simulink model "EHB_speedgoat_R2020a_V1"  (R2020a)
settings: Solver=FixedStepDiscrete  StartTime=0.0  StopTime=inf  FixedStep=0.001  RelTol=1e-3  EnableMultiTasking=on
model workspace (MAT data in the model file):
  A : Simulink.Signal (value not decoded)
  B : Simulink.Signal (value not decoded)
  C : Simulink.Signal (value not decoded)
  D : Simulink.Signal (value not decoded)
  E : Simulink.Signal (value not decoded)
  calin = [-9.96 -7.98 -5.98 -3.99 -1.994 0 1.995 3.992 5.99 7.98 9.97]
  calout = [-10 -8 -6 -4 -2 0 2 4 6 8 10]
symbols that are objects in the model workspace (value not decoded): C, D
undefined symbols (not defined in the file): Com1, none, ts_IO612
libraries: simulink x1436, xpcethercatlib x1223, yisutbxlib_utilities x256, xpcutilitieslib x156, hdlsllib x145, canmsglib x46, speedgoatlib_IO602_4 x11, speedgoatlib_IO611 x7, slrttcplib x4, CanManageLib x3, slrtlib x3, xpcseriallib x2
(part 25 of 30)

== system EHB_speedgoat_R2020a_V1/保留/YS4008/YS4008_M_5/YS4008_M/FIU_MsgSend ==
  YS4008_M : Inport
  Enable : EnablePort
  Bus Selector : BusSelector  OutputSignals=CH1_Out.KL30_Out,CH1_Out.KL31_Out,CH1_Out.COM_Out,CH1_Out.Open_Out,CH2_Out.KL30_Out,CH2_Out.KL31_Out,CH2_Out.COM_Out,CH2_Out.Open_Out,CH3_Out.KL30_Out,CH3_Out.KL31_Out,CH3_Out.COM_Out,CH3_Out.Open_Out,CH4_Out.KL30_Out,CH4_Out.KL31_Out,CH4_Out.COM_Out,CH4_Out.Open_Out,CH5_Out.KL30_Out,CH5_Out.KL31_Out,CH5_Out.COM_Out,CH5_Out.Open_Out,CH6_Out.KL30_Out,CH6_Out.KL31_Out,CH6_Out.COM_Out,CH6_Out.Open_Out,CH7_Out.KL30_Out,CH7_Out.KL31_Out,CH7_Out.COM_Out,CH7_Out.Open_Out,CH8_Out.KL30_Out,CH8_Out.KL31_Out,CH8_Out.COM_Out,CH8_Out.Open_Out,PassWord,Rack,Slot
  CAN Pack8 : canmsglib/CAN Pack  MsgList=(none)  MsgName=FIUStsSet  MsgIDType=Standard (11-bit identifier)  MsgIdentifier=1669  MsgLength=8  Remote=off  ApplyMinMax=off  BusOutput=on  SignalInfo={ 'CH1_COM', '26', '1', 'BE', 'unsigned', 'Standard', '0', '1', '0', '0', '1'; 'CH1_KL30', '24', '1', 'BE', 'unsigned', 'Standard', '0', '1', '0', '0', '1'; 'CH1_KL31', '25', '1', 'BE', 'unsigned', 'Standard', '0', '1', '0', '0', '1'; 'CH1_Open', '27', '1', 'BE', 'unsigned', 'Standard', '0', '1', '0', '0', '1'; 'CH2_COM', '30', '1', 'BE', 'unsigned', 'Standard', '0', '1', '0', '0', '1'; 'CH2_KL30', '28', '1', 'BE', 'unsigned', 'Standard', '0', '1', '0', '0', '1'; 'CH2_KL31', '29', '1', 'BE', 'unsigned', 'Standard', '0', '1', '0', '0', '1'; 'CH2_Open', '31', '1', 'BE', 'unsigned', 'Standard', '0', '1', '0', '0', '1'; 'CH3_COM', '34', '1', 'BE', 'unsigned', 'Standard', '0', '1', '0', '0', '1'; 'CH3_KL30', '32', '1', 'BE', 'unsigned', 'Standard', '0', '1', '0', '0', '1'; 'CH3_KL31', '33', '1', 'BE', 'unsigned', 'Standard', '0', '1', '0', '0', '1'; 'CH3_Open', '35', '1', 'BE', 'unsigned', 'Standard', '0', '1', '0', '0', '1'; 'CH4_COM', '38', '1', 'BE', 'unsigned', 'Standard', '0', '1', '0', '0', '1'; 'CH4_KL30', '36', '1', 'BE', 'unsigned', 'Standard', '0', '1', '0', '0', '1'; 'CH4_KL31', '37', '1', 'BE', 'unsigned', 'Standard', '0', '1', '0', '0', '1'; 'CH4_Open', '39', '1', 'BE', 'unsigned', 'Standard', '0', '1', '0', '0', '1'; 'CH5_COM', '42', '1', 'BE', 'unsigned', 'Standard', '0', '1', '0', '0', '1'; 'CH5_KL30', '40', '1', 'BE', 'unsigned', 'Standard', '0', '1', '0', '0', '1'; 'CH5_KL31', '41', '1', 'BE', 'unsigned', 'Standard', '0', '1', '0', '0', '1'; 'CH5_Open', '43', '1', 'BE', 'unsigned', 'Standard', '0', '1', '0', '0', '1'; 'CH6_COM', '46', '1', 'BE', 'unsigned', 'Standard', '0', '1', '0', '0', '1'; 'CH6_KL30', '44', '1', 'BE', 'unsigned', 'Standard', '0', '1', '0', '0', '1'; 'CH6_KL31', '45', '1', 'BE', 'unsigned', 'Standard', '0', '1', '0', '0', '1'; 'CH6_Open', '47', '1', 'BE', 'unsigned', 'Standard', '0', '1', '0', '0', '1'; 'CH7_COM', '50', '1', 'BE', 'unsigned', 'Standard', '0', '1', '0', '0', '1'; 'CH7_KL30', '48', '1', 'BE', 'unsigned', 'Standard', '0', '1', '0', '0', '1'; 'CH7_KL31', '49', '1', 'BE', 'unsigned', 'Standard', '0', '1', '0', '0', '1'; 'CH7_Open', '51', '1', 'BE', 'unsigned', 'Standard', '0', '1', '0', '0', '1'; 'CH8_COM', '54', '1', 'BE', 'unsigned', 'Standard', '0', '1', '0', '0', '1'; 'CH8_KL30', '52', '1', 'BE', 'unsigned', 'Standard', '0', '1', '0', '0', '1'; 'CH8_KL31', '53', '1', 'BE', 'unsigned', 'Standard', '0', '1', '0', '0', '1'; 'CH8_Open', '55', '1', 'BE', 'unsigned', 'Standard', '0', '1', '0', '0', '1'; 'Password', '16', '8', 'BE', 'unsigned', 'Standard', '0', '1', '0', '0', '15'; 'Rack', '0', '4', 'BE', 'signed', 'Standard', '0', '1', '0', '-Inf', 'Inf'; 'Slot', '4', '4', 'BE', 'signed', 'Standard', '0', '1', '0', '-Inf', 'Inf' }
      settings: SourceProductBaseCode=XP,ME,VN  DataFormat=manually specified signals
  CANDataPack_ToUDP : Subsystem
  Output : Outport
  wires:
  YS4008_M/1 -> Bus Selector/1
  [CH1_COM] -> CAN Pack8/1  "CH1_COM"
  [CH1_KL30] -> CAN Pack8/2  "CH1_KL30"
  [CH1_KL31] -> CAN Pack8/3  "CH1_KL31"
  [CH1_Open] -> CAN Pack8/4  "CH1_Open"
  [CH2_COM] -> CAN Pack8/5  "CH2_COM"
  [CH2_KL30] -> CAN Pack8/6  "CH2_KL30"
  [CH2_KL31] -> CAN Pack8/7  "CH2_KL31"
  [CH2_Open] -> CAN Pack8/8  "CH2_Open"
  [CH3_COM] -> CAN Pack8/9  "CH3_COM"
  [CH3_KL30] -> CAN Pack8/10  "CH3_KL30"
  [CH3_KL31] -> CAN Pack8/11  "CH3_KL31"
  [CH3_Open] -> CAN Pack8/12  "CH3_Open"
  [CH4_COM] -> CAN Pack8/13  "CH4_COM"
  [CH4_KL30] -> CAN Pack8/14  "CH4_KL30"
  [CH4_KL31] -> CAN Pack8/15  "CH4_KL31"
  [CH4_Open] -> CAN Pack8/16  "CH4_Open"
  [CH5_COM] -> CAN Pack8/17  "CH5_COM"
  [CH5_KL30] -> CAN Pack8/18  "CH5_KL30"
  [CH5_KL31] -> CAN Pack8/19  "CH5_KL31"
  [CH5_Open] -> CAN Pack8/20  "CH5_Open"
  [CH6_COM] -> CAN Pack8/21  "CH6_COM"
  [CH6_KL30] -> CAN Pack8/22  "CH6_KL30"
  [CH6_KL31] -> CAN Pack8/23  "CH6_KL31"
  [CH6_Open] -> CAN Pack8/24  "CH6_Open"
  [CH7_COM] -> CAN Pack8/25  "CH7_COM"
  [CH7_KL30] -> CAN Pack8/26  "CH7_KL30"
  [CH7_KL31] -> CAN Pack8/27  "CH7_KL31"
  [CH7_Open] -> CAN Pack8/28  "CH7_Open"
  [CH8_COM] -> CAN Pack8/29  "CH8_COM"
  [CH8_KL30] -> CAN Pack8/30  "CH8_KL30"
  [CH8_KL31] -> CAN Pack8/31  "CH8_KL31"
  [CH8_Open] -> CAN Pack8/32  "CH8_Open"
  [PassWord] -> CAN Pack8/33  "PassWord"
  Bus Selector/33 -> [PassWord]  "<PassWord>"
  Bus Selector/9 -> [CH3_KL30]  "<KL30_Out>"
  Bus Selector/10 -> [CH3_KL31]  "<KL31_Out>"
  Bus Selector/11 -> [CH3_COM]  "<COM_Out>"
  Bus Selector/12 -> [CH3_Open]  "<Open_Out>"
  Bus Selector/13 -> [CH4_KL30]  "<KL30_Out>"
  Bus Selector/14 -> [CH4_KL31]  "<KL31_Out>"
  Bus Selector/15 -> [CH4_COM]  "<COM_Out>"
  Bus Selector/16 -> [CH4_Open]  "<Open_Out>"
  Bus Selector/17 -> [CH5_KL30]  "<KL30_Out>"
  Bus Selector/18 -> [CH5_KL31]  "<KL31_Out>"
  Bus Selector/19 -> [CH5_COM]  "<COM_Out>"
  Bus Selector/20 -> [CH5_Open]  "<Open_Out>"
  Bus Selector/21 -> [CH6_KL30]  "<KL30_Out>"
  Bus Selector/22 -> [CH6_KL31]  "<KL31_Out>"
  Bus Selector/23 -> [CH6_COM]  "<COM_Out>"
  Bus Selector/24 -> [CH6_Open]  "<Open_Out>"
  Bus Selector/25 -> [CH7_KL30]  "<KL30_Out>"
  Bus Selector/26 -> [CH7_KL31]  "<KL31_Out>"
  Bus Selector/27 -> [CH7_COM]  "<COM_Out>"
  Bus Selector/28 -> [CH7_Open]  "<Open_Out>"
  Bus Selector/29 -> [CH8_KL30]  "<KL30_Out>"
  Bus Selector/30 -> [CH8_KL31]  "<KL31_Out>"
  Bus Selector/31 -> [CH8_COM]  "<COM_Out>"
  Bus Selector/32 -> [CH8_Open]  "<Open_Out>"
  Bus Selector/1 -> [CH1_KL30]  "<KL30_Out>"
  Bus Selector/2 -> [CH1_KL31]  "<KL31_Out>"
  Bus Selector/3 -> [CH1_COM]  "<COM_Out>"
  Bus Selector/4 -> [CH1_Open]  "<Open_Out>"
  Bus Selector/5 -> [CH2_KL30]  "<KL30_Out>"
  Bus Selector/6 -> [CH2_KL31]  "<KL31_Out>"
  Bus Selector/7 -> [CH2_COM]  "<COM_Out>"
  Bus Selector/8 -> [CH2_Open]  "<Open_Out>"
  [Rack] -> CAN Pack8/34  "Rack"
  [Slot] -> CAN Pack8/35  "Slot"
  Bus Selector/34 -> [Rack]  "<Rack>"
  Bus Selector/35 -> [Slot]  "<Slot>"
  CAN Pack8/1 -> CANDataPack_ToUDP/1(In1)
  CANDataPack_ToUDP/1(Output) -> Output/1

== system EHB_speedgoat_R2020a_V1/保留/YS4008/YS4008_M_5/YS4008_M/YS4008_M_Ctrl_Trigger ==
  YS4008_M : Inport
  Bitwise Operator : simulink/Logic and Bit Operations/Bitwise Operator  logicop=OR  UseBitMask=off  BitMask=bin2dec('11011001')  BitMaskRealWorld=Stored Integer
  Bus Selector : BusSelector  OutputSignals=FIU_SetCH1,FIU_SetCH2,FIU_SetCH3,FIU_SetCH4,FIU_SetCH5,FIU_SetCH6,FIU_SetCH7,FIU_SetCH8
  Detect Change : simulink/Logic and Bit Operations/Detect Change  vinit=0  OutDataTypeStr=boolean
  Mux : Mux  Inputs=8
  YS4008_M_CtrlTrigger : Outport
  wires:
  Detect Change/1 -> Bitwise Operator/1
  Mux/1 -> Detect Change/1
  Bitwise Operator/1 -> YS4008_M_CtrlTrigger/1
  YS4008_M/1 -> Bus Selector/1
  Bus Selector/1 -> Mux/1  "<FIU_SetCH1>"
  Bus Selector/2 -> Mux/2  "<FIU_SetCH2>"
  Bus Selector/3 -> Mux/3  "<FIU_SetCH3>"
  Bus Selector/4 -> Mux/4  "<FIU_SetCH4>"
  Bus Selector/5 -> Mux/5  "<FIU_SetCH5>"
  Bus Selector/6 -> Mux/6  "<FIU_SetCH6>"
  Bus Selector/7 -> Mux/7  "<FIU_SetCH7>"
  Bus Selector/8 -> Mux/8  "<FIU_SetCH8>"

== system EHB_speedgoat_R2020a_V1/保留/YS4008/YS4008_M_6/YS4008_M/FIU_CH1 ==
  FIU_SetCH1 : Inport
  Bit Unpacking 1 : xpcutilitieslib/Bit Unpacking   SignExtend=on  MaskBitPatterns={[0],[1],[2],[3]}  MaskPackDataType=uint8  MaskPackDataSize=[1]  MaskUnpackDataTypes={'boolean','boolean','boolean','boolean'}  MaskUnpackDataSizes={[1],[1],[1],[1]}
      settings: SourceProductBaseCode=XP
  Bus Creator : BusCreator  Inputs=4
  Protect : Subsystem
  CH1_Out : Outport
  wires:
  FIU_SetCH1/1 -> Bit Unpacking 1/1
  Protect/3(COM_Out) -> Bus Creator/3  "COM_Out"
  Protect/2(KL31_Out) -> Bus Creator/2  "KL31_Out"
  Protect/1(KL30_Out) -> Bus Creator/1  "KL30_Out"
  Protect/4(Open_Out) -> Bus Creator/4  "Open_Out"
  Bit Unpacking 1/1 -> Protect/1(KL30_In)
  Bit Unpacking 1/2 -> Protect/2(KL31_In)
  Bit Unpacking 1/3 -> Protect/3(COM_In)
  Bit Unpacking 1/4 -> Protect/4(Open_In)
  Bus Creator/1 -> CH1_Out/1

== system EHB_speedgoat_R2020a_V1/保留/YS4008/YS4008_M_6/YS4008_M/FIU_CH2 ==
  FIU_SetCH2 : Inport
  Bit Unpacking 1 : xpcutilitieslib/Bit Unpacking   SignExtend=on  MaskBitPatterns={[0],[1],[2],[3]}  MaskPackDataType=uint8  MaskPackDataSize=[1]  MaskUnpackDataTypes={'boolean','boolean','boolean','boolean'}  MaskUnpackDataSizes={[1],[1],[1],[1]}
      settings: SourceProductBaseCode=XP
  Bus Creator : BusCreator  Inputs=4
  Protect : Subsystem
  CH2_Out : Outport
  wires:
  Bus Creator/1 -> CH2_Out/1
  Bit Unpacking 1/4 -> Protect/4(Open_In)
  Bit Unpacking 1/3 -> Protect/3(COM_In)
  Bit Unpacking 1/2 -> Protect/2(KL31_In)
  Bit Unpacking 1/1 -> Protect/1(KL30_In)
  Protect/4(Open_Out) -> Bus Creator/4  "Open_Out"
  Protect/1(KL30_Out) -> Bus Creator/1  "KL30_Out"
  Protect/2(KL31_Out) -> Bus Creator/2  "KL31_Out"
  Protect/3(COM_Out) -> Bus Creator/3  "COM_Out"
  FIU_SetCH2/1 -> Bit Unpacking 1/1

== system EHB_speedgoat_R2020a_V1/保留/YS4008/YS4008_M_6/YS4008_M/FIU_CH3 ==
  FIU_SetCH3 : Inport
  Bit Unpacking 1 : xpcutilitieslib/Bit Unpacking   SignExtend=on  MaskBitPatterns={[0],[1],[2],[3]}  MaskPackDataType=uint8  MaskPackDataSize=[1]  MaskUnpackDataTypes={'boolean','boolean','boolean','boolean'}  MaskUnpackDataSizes={[1],[1],[1],[1]}
      settings: SourceProductBaseCode=XP
  Bus Creator : BusCreator  Inputs=4
  Protect : Subsystem
  CH3_Out : Outport
  wires:
  FIU_SetCH3/1 -> Bit Unpacking 1/1
  Protect/3(COM_Out) -> Bus Creator/3  "COM_Out"
  Protect/2(KL31_Out) -> Bus Creator/2  "KL31_Out"
  Protect/1(KL30_Out) -> Bus Creator/1  "KL30_Out"
  Protect/4(Open_Out) -> Bus Creator/4  "Open_Out"
  Bit Unpacking 1/1 -> Protect/1(KL30_In)
  Bit Unpacking 1/2 -> Protect/2(KL31_In)
  Bit Unpacking 1/3 -> Protect/3(COM_In)
  Bit Unpacking 1/4 -> Protect/4(Open_In)
  Bus Creator/1 -> CH3_Out/1

== system EHB_speedgoat_R2020a_V1/保留/YS4008/YS4008_M_6/YS4008_M/FIU_CH4 ==
  FIU_SetCH4 : Inport
  Bit Unpacking 1 : xpcutilitieslib/Bit Unpacking   SignExtend=on  MaskBitPatterns={[0],[1],[2],[3]}  MaskPackDataType=uint8  MaskPackDataSize=[1]  MaskUnpackDataTypes={'boolean','boolean','boolean','boolean'}  MaskUnpackDataSizes={[1],[1],[1],[1]}
      settings: SourceProductBaseCode=XP
  Bus Creator : BusCreator  Inputs=4
  Protect : Subsystem
  CH4_Out : Outport
  wires:
  Bus Creator/1 -> CH4_Out/1
  Bit Unpacking 1/4 -> Protect/4(Open_In)
  Bit Unpacking 1/3 -> Protect/3(COM_In)
  Bit Unpacking 1/2 -> Protect/2(KL31_In)
  Bit Unpacking 1/1 -> Protect/1(KL30_In)
  Protect/4(Open_Out) -> Bus Creator/4  "Open_Out"
  Protect/1(KL30_Out) -> Bus Creator/1  "KL30_Out"
  Protect/2(KL31_Out) -> Bus Creator/2  "KL31_Out"
  Protect/3(COM_Out) -> Bus Creator/3  "COM_Out"
  FIU_SetCH4/1 -> Bit Unpacking 1/1

== system EHB_speedgoat_R2020a_V1/保留/YS4008/YS4008_M_6/YS4008_M/FIU_CH5 ==
  FIU_SetCH5 : Inport
  Bit Unpacking 1 : xpcutilitieslib/Bit Unpacking   SignExtend=on  MaskBitPatterns={[0],[1],[2],[3]}  MaskPackDataType=uint8  MaskPackDataSize=[1]  MaskUnpackDataTypes={'boolean','boolean','boolean','boolean'}  MaskUnpackDataSizes={[1],[1],[1],[1]}
      settings: SourceProductBaseCode=XP
  Bus Creator : BusCreator  Inputs=4
  Protect : Subsystem
  CH5_Out : Outport
  wires:
  FIU_SetCH5/1 -> Bit Unpacking 1/1
  Protect/3(COM_Out) -> Bus Creator/3  "COM_Out"
  Protect/2(KL31_Out) -> Bus Creator/2  "KL31_Out"
  Protect/1(KL30_Out) -> Bus Creator/1  "KL30_Out"
  Protect/4(Open_Out) -> Bus Creator/4  "Open_Out"
  Bit Unpacking 1/1 -> Protect/1(KL30_In)
  Bit Unpacking 1/2 -> Protect/2(KL31_In)
  Bit Unpacking 1/3 -> Protect/3(COM_In)
  Bit Unpacking 1/4 -> Protect/4(Open_In)
  Bus Creator/1 -> CH5_Out/1

== system EHB_speedgoat_R2020a_V1/保留/YS4008/YS4008_M_6/YS4008_M/FIU_CH6 ==
  FIU_SetCH6 : Inport
  Bit Unpacking 1 : xpcutilitieslib/Bit Unpacking   SignExtend=on  MaskBitPatterns={[0],[1],[2],[3]}  MaskPackDataType=uint8  MaskPackDataSize=[1]  MaskUnpackDataTypes={'boolean','boolean','boolean','boolean'}  MaskUnpackDataSizes={[1],[1],[1],[1]}
      settings: SourceProductBaseCode=XP
  Bus Creator : BusCreator  Inputs=4
  Protect : Subsystem
  CH6_Out : Outport
  wires:
  Bus Creator/1 -> CH6_Out/1
  Bit Unpacking 1/4 -> Protect/4(Open_In)
  Bit Unpacking 1/3 -> Protect/3(COM_In)
  Bit Unpacking 1/2 -> Protect/2(KL31_In)
  Bit Unpacking 1/1 -> Protect/1(KL30_In)
  Protect/4(Open_Out) -> Bus Creator/4  "Open_Out"
  Protect/1(KL30_Out) -> Bus Creator/1  "KL30_Out"
  Protect/2(KL31_Out) -> Bus Creator/2  "KL31_Out"
  Protect/3(COM_Out) -> Bus Creator/3  "COM_Out"
  FIU_SetCH6/1 -> Bit Unpacking 1/1

== system EHB_speedgoat_R2020a_V1/保留/YS4008/YS4008_M_6/YS4008_M/FIU_CH7 ==
  FIU_SetCH7 : Inport
  Bit Unpacking 1 : xpcutilitieslib/Bit Unpacking   SignExtend=on  MaskBitPatterns={[0],[1],[2],[3]}  MaskPackDataType=uint8  MaskPackDataSize=[1]  MaskUnpackDataTypes={'boolean','boolean','boolean','boolean'}  MaskUnpackDataSizes={[1],[1],[1],[1]}
      settings: SourceProductBaseCode=XP
  Bus Creator : BusCreator  Inputs=4
  Protect : Subsystem
  CH7_Out : Outport
  wires:
  FIU_SetCH7/1 -> Bit Unpacking 1/1
  Protect/3(COM_Out) -> Bus Creator/3  "COM_Out"
  Protect/2(KL31_Out) -> Bus Creator/2  "KL31_Out"
  Protect/1(KL30_Out) -> Bus Creator/1  "KL30_Out"
  Protect/4(Open_Out) -> Bus Creator/4  "Open_Out"
  Bit Unpacking 1/1 -> Protect/1(KL30_In)
  Bit Unpacking 1/2 -> Protect/2(KL31_In)
  Bit Unpacking 1/3 -> Protect/3(COM_In)
  Bit Unpacking 1/4 -> Protect/4(Open_In)
  Bus Creator/1 -> CH7_Out/1

== system EHB_speedgoat_R2020a_V1/保留/YS4008/YS4008_M_6/YS4008_M/FIU_CH8 ==
  FIU_SetCH8 : Inport
  Bit Unpacking 1 : xpcutilitieslib/Bit Unpacking   SignExtend=on  MaskBitPatterns={[0],[1],[2],[3]}  MaskPackDataType=uint8  MaskPackDataSize=[1]  MaskUnpackDataTypes={'boolean','boolean','boolean','boolean'}  MaskUnpackDataSizes={[1],[1],[1],[1]}
      settings: SourceProductBaseCode=XP
  Bus Creator : BusCreator  Inputs=4
  Protect : Subsystem
  CH8_Out : Outport
  wires:
  Bus Creator/1 -> CH8_Out/1
  Bit Unpacking 1/4 -> Protect/4(Open_In)
  Bit Unpacking 1/3 -> Protect/3(COM_In)
  Bit Unpacking 1/2 -> Protect/2(KL31_In)
  Bit Unpacking 1/1 -> Protect/1(KL30_In)
  Protect/4(Open_Out) -> Bus Creator/4  "Open_Out"
  Protect/1(KL30_Out) -> Bus Creator/1  "KL30_Out"
  Protect/2(KL31_Out) -> Bus Creator/2  "KL31_Out"
  Protect/3(COM_Out) -> Bus Creator/3  "COM_Out"
  FIU_SetCH8/1 -> Bit Unpacking 1/1

== system EHB_speedgoat_R2020a_V1/保留/YS4008/YS4008_M_6/YS4008_M/FIU_MsgSend ==
  YS4008_M : Inport
  Enable : EnablePort
  Bus Selector : BusSelector  OutputSignals=CH1_Out.KL30_Out,CH1_Out.KL31_Out,CH1_Out.COM_Out,CH1_Out.Open_Out,CH2_Out.KL30_Out,CH2_Out.KL31_Out,CH2_Out.COM_Out,CH2_Out.Open_Out,CH3_Out.KL30_Out,CH3_Out.KL31_Out,CH3_Out.COM_Out,CH3_Out.Open_Out,CH4_Out.KL30_Out,CH4_Out.KL31_Out,CH4_Out.COM_Out,CH4_Out.Open_Out,CH5_Out.KL30_Out,CH5_Out.KL31_Out,CH5_Out.COM_Out,CH5_Out.Open_Out,CH6_Out.KL30_Out,CH6_Out.KL31_Out,CH6_Out.COM_Out,CH6_Out.Open_Out,CH7_Out.KL30_Out,CH7_Out.KL31_Out,CH7_Out.COM_Out,CH7_Out.Open_Out,CH8_Out.KL30_Out,CH8_Out.KL31_Out,CH8_Out.COM_Out,CH8_Out.Open_Out,PassWord,Rack,Slot
  CAN Pack8 : canmsglib/CAN Pack  MsgList=(none)  MsgName=FIUStsSet  MsgIDType=Standard (11-bit identifier)  MsgIdentifier=1670  MsgLength=8  Remote=off  ApplyMinMax=off  BusOutput=on  SignalInfo={ 'CH1_COM', '26', '1', 'BE', 'unsigned', 'Standard', '0', '1', '0', '0', '1'; 'CH1_KL30', '24', '1', 'BE', 'unsigned', 'Standard', '0', '1', '0', '0', '1'; 'CH1_KL31', '25', '1', 'BE', 'unsigned', 'Standard', '0', '1', '0', '0', '1'; 'CH1_Open', '27', '1', 'BE', 'unsigned', 'Standard', '0', '1', '0', '0', '1'; 'CH2_COM', '30', '1', 'BE', 'unsigned', 'Standard', '0', '1', '0', '0', '1'; 'CH2_KL30', '28', '1', 'BE', 'unsigned', 'Standard', '0', '1', '0', '0', '1'; 'CH2_KL31', '29', '1', 'BE', 'unsigned', 'Standard', '0', '1', '0', '0', '1'; 'CH2_Open', '31', '1', 'BE', 'unsigned', 'Standard', '0', '1', '0', '0', '1'; 'CH3_COM', '34', '1', 'BE', 'unsigned', 'Standard', '0', '1', '0', '0', '1'; 'CH3_KL30', '32', '1', 'BE', 'unsigned', 'Standard', '0', '1', '0', '0', '1'; 'CH3_KL31', '33', '1', 'BE', 'unsigned', 'Standard', '0', '1', '0', '0', '1'; 'CH3_Open', '35', '1', 'BE', 'unsigned', 'Standard', '0', '1', '0', '0', '1'; 'CH4_COM', '38', '1', 'BE', 'unsigned', 'Standard', '0', '1', '0', '0', '1'; 'CH4_KL30', '36', '1', 'BE', 'unsigned', 'Standard', '0', '1', '0', '0', '1'; 'CH4_KL31', '37', '1', 'BE', 'unsigned', 'Standard', '0', '1', '0', '0', '1'; 'CH4_Open', '39', '1', 'BE', 'unsigned', 'Standard', '0', '1', '0', '0', '1'; 'CH5_COM', '42', '1', 'BE', 'unsigned', 'Standard', '0', '1', '0', '0', '1'; 'CH5_KL30', '40', '1', 'BE', 'unsigned', 'Standard', '0', '1', '0', '0', '1'; 'CH5_KL31', '41', '1', 'BE', 'unsigned', 'Standard', '0', '1', '0', '0', '1'; 'CH5_Open', '43', '1', 'BE', 'unsigned', 'Standard', '0', '1', '0', '0', '1'; 'CH6_COM', '46', '1', 'BE', 'unsigned', 'Standard', '0', '1', '0', '0', '1'; 'CH6_KL30', '44', '1', 'BE', 'unsigned', 'Standard', '0', '1', '0', '0', '1'; 'CH6_KL31', '45', '1', 'BE', 'unsigned', 'Standard', '0', '1', '0', '0', '1'; 'CH6_Open', '47', '1', 'BE', 'unsigned', 'Standard', '0', '1', '0', '0', '1'; 'CH7_COM', '50', '1', 'BE', 'unsigned', 'Standard', '0', '1', '0', '0', '1'; 'CH7_KL30', '48', '1', 'BE', 'unsigned', 'Standard', '0', '1', '0', '0', '1'; 'CH7_KL31', '49', '1', 'BE', 'unsigned', 'Standard', '0', '1', '0', '0', '1'; 'CH7_Open', '51', '1', 'BE', 'unsigned', 'Standard', '0', '1', '0', '0', '1'; 'CH8_COM', '54', '1', 'BE', 'unsigned', 'Standard', '0', '1', '0', '0', '1'; 'CH8_KL30', '52', '1', 'BE', 'unsigned', 'Standard', '0', '1', '0', '0', '1'; 'CH8_KL31', '53', '1', 'BE', 'unsigned', 'Standard', '0', '1', '0', '0', '1'; 'CH8_Open', '55', '1', 'BE', 'unsigned', 'Standard', '0', '1', '0', '0', '1'; 'Password', '16', '8', 'BE', 'unsigned', 'Standard', '0', '1', '0', '0', '15'; 'Rack', '0', '4', 'BE', 'signed', 'Standard', '0', '1', '0', '-Inf', 'Inf'; 'Slot', '4', '4', 'BE', 'signed', 'Standard', '0', '1', '0', '-Inf', 'Inf' }
      settings: SourceProductBaseCode=XP,ME,VN  DataFormat=manually specified signals
  CANDataPack_ToUDP : Subsystem
  Output : Outport
  wires:
  YS4008_M/1 -> Bus Selector/1
  [CH1_COM] -> CAN Pack8/1  "CH1_COM"
  [CH1_KL30] -> CAN Pack8/2  "CH1_KL30"
  [CH1_KL31] -> CAN Pack8/3  "CH1_KL31"
  [CH1_Open] -> CAN Pack8/4  "CH1_Open"
  [CH2_COM] -> CAN Pack8/5  "CH2_COM"
  [CH2_KL30] -> CAN Pack8/6  "CH2_KL30"
  [CH2_KL31] -> CAN Pack8/7  "CH2_KL31"
  [CH2_Open] -> CAN Pack8/8  "CH2_Open"
  [CH3_COM] -> CAN Pack8/9  "CH3_COM"
  [CH3_KL30] -> CAN Pack8/10  "CH3_KL30"
  [CH3_KL31] -> CAN Pack8/11  "CH3_KL31"
  [CH3_Open] -> CAN Pack8/12  "CH3_Open"
  [CH4_COM] -> CAN Pack8/13  "CH4_COM"
  [CH4_KL30] -> CAN Pack8/14  "CH4_KL30"
  [CH4_KL31] -> CAN Pack8/15  "CH4_KL31"
  [CH4_Open] -> CAN Pack8/16  "CH4_Open"
  [CH5_COM] -> CAN Pack8/17  "CH5_COM"
  [CH5_KL30] -> CAN Pack8/18  "CH5_KL30"
  [CH5_KL31] -> CAN Pack8/19  "CH5_KL31"
  [CH5_Open] -> CAN Pack8/20  "CH5_Open"
  [CH6_COM] -> CAN Pack8/21  "CH6_COM"
  [CH6_KL30] -> CAN Pack8/22  "CH6_KL30"
  [CH6_KL31] -> CAN Pack8/23  "CH6_KL31"
  [CH6_Open] -> CAN Pack8/24  "CH6_Open"
  [CH7_COM] -> CAN Pack8/25  "CH7_COM"
  [CH7_KL30] -> CAN Pack8/26  "CH7_KL30"
  [CH7_KL31] -> CAN Pack8/27  "CH7_KL31"
  [CH7_Open] -> CAN Pack8/28  "CH7_Open"
  [CH8_COM] -> CAN Pack8/29  "CH8_COM"
  [CH8_KL30] -> CAN Pack8/30  "CH8_KL30"
  [CH8_KL31] -> CAN Pack8/31  "CH8_KL31"
  [CH8_Open] -> CAN Pack8/32  "CH8_Open"
  [PassWord] -> CAN Pack8/33  "PassWord"
  Bus Selector/33 -> [PassWord]  "<PassWord>"
  Bus Selector/9 -> [CH3_KL30]  "<KL30_Out>"
  Bus Selector/10 -> [CH3_KL31]  "<KL31_Out>"
  Bus Selector/11 -> [CH3_COM]  "<COM_Out>"
  Bus Selector/12 -> [CH3_Open]  "<Open_Out>"
  Bus Selector/13 -> [CH4_KL30]  "<KL30_Out>"
  Bus Selector/14 -> [CH4_KL31]  "<KL31_Out>"
  Bus Selector/15 -> [CH4_COM]  "<COM_Out>"
  Bus Selector/16 -> [CH4_Open]  "<Open_Out>"
  Bus Selector/17 -> [CH5_KL30]  "<KL30_Out>"
  Bus Selector/18 -> [CH5_KL31]  "<KL31_Out>"
  Bus Selector/19 -> [CH5_COM]  "<COM_Out>"
  Bus Selector/20 -> [CH5_Open]  "<Open_Out>"
  Bus Selector/21 -> [CH6_KL30]  "<KL30_Out>"
  Bus Selector/22 -> [CH6_KL31]  "<KL31_Out>"
  Bus Selector/23 -> [CH6_COM]  "<COM_Out>"
  Bus Selector/24 -> [CH6_Open]  "<Open_Out>"
  Bus Selector/25 -> [CH7_KL30]  "<KL30_Out>"
  Bus Selector/26 -> [CH7_KL31]  "<KL31_Out>"
  Bus Selector/27 -> [CH7_COM]  "<COM_Out>"
  Bus Selector/28 -> [CH7_Open]  "<Open_Out>"
  Bus Selector/29 -> [CH8_KL30]  "<KL30_Out>"
  Bus Selector/30 -> [CH8_KL31]  "<KL31_Out>"
  Bus Selector/31 -> [CH8_COM]  "<COM_Out>"
  Bus Selector/32 -> [CH8_Open]  "<Open_Out>"
  Bus Selector/1 -> [CH1_KL30]  "<KL30_Out>"
  Bus Selector/2 -> [CH1_KL31]  "<KL31_Out>"
  Bus Selector/3 -> [CH1_COM]  "<COM_Out>"
  Bus Selector/4 -> [CH1_Open]  "<Open_Out>"
  Bus Selector/5 -> [CH2_KL30]  "<KL30_Out>"
  Bus Selector/6 -> [CH2_KL31]  "<KL31_Out>"
  Bus Selector/7 -> [CH2_COM]  "<COM_Out>"
  Bus Selector/8 -> [CH2_Open]  "<Open_Out>"
  [Rack] -> CAN Pack8/34  "Rack"
  [Slot] -> CAN Pack8/35  "Slot"
  Bus Selector/34 -> [Rack]  "<Rack>"
  Bus Selector/35 -> [Slot]  "<Slot>"
  CAN Pack8/1 -> CANDataPack_ToUDP/1(In1)
  CANDataPack_ToUDP/1(Output) -> Output/1

== system EHB_speedgoat_R2020a_V1/保留/YS4008/YS4008_M_6/YS4008_M/YS4008_M_Ctrl_Trigger ==
  YS4008_M : Inport
  Bitwise Operator : simulink/Logic and Bit Operations/Bitwise Operator  logicop=OR  UseBitMask=off  BitMask=bin2dec('11011001')  BitMaskRealWorld=Stored Integer
  Bus Selector : BusSelector  OutputSignals=FIU_SetCH1,FIU_SetCH2,FIU_SetCH3,FIU_SetCH4,FIU_SetCH5,FIU_SetCH6,FIU_SetCH7,FIU_SetCH8
  Detect Change : simulink/Logic and Bit Operations/Detect Change  vinit=0  OutDataTypeStr=boolean
  Mux : Mux  Inputs=8
  YS4008_M_CtrlTrigger : Outport
  wires:
  Detect Change/1 -> Bitwise Operator/1
  Mux/1 -> Detect Change/1
  Bitwise Operator/1 -> YS4008_M_CtrlTrigger/1
  YS4008_M/1 -> Bus Selector/1
  Bus Selector/1 -> Mux/1  "<FIU_SetCH1>"
  Bus Selector/2 -> Mux/2  "<FIU_SetCH2>"
  Bus Selector/3 -> Mux/3  "<FIU_SetCH3>"
  Bus Selector/4 -> Mux/4  "<FIU_SetCH4>"
  Bus Selector/5 -> Mux/5  "<FIU_SetCH5>"
  Bus Selector/6 -> Mux/6  "<FIU_SetCH6>"
  Bus Selector/7 -> Mux/7  "<FIU_SetCH7>"
  Bus Selector/8 -> Mux/8  "<FIU_SetCH8>"

== system EHB_speedgoat_R2020a_V1/CAN_Send/Trigger/Trigger_VCU_Msg/Trigger_VCU_BrakingRequest_0x120/Cycle/Triggered Subsystem1 ==
  SendFlag : Inport
  MsgLstCnt : Inport  Port=2
  Enable : EnablePort
  Add : Sum
  Constant1 : Constant  Value=0  SampleTime=-1
  Data Type Conversion : DataTypeConversion
  Data Type Conversion1 : DataTypeConversion
  Delay : Delay  DelayLength=1  ExternalReset=Rising
      settings: InputPortMap=u0,r5
  Delay2 : Delay  DelayLength=1
  Relational Operator : RelationalOperator  Operator=>  OutDataTypeStr=boolean  RndMeth=Simplest
  Relational Operator1 : RelationalOperator  Operator=~=  OutDataTypeStr=boolean  RndMeth=Simplest
  Switch : Switch  Criteria=u2 > Threshold
  Out1 : Outport  OutputWhenDisabled=reset  InitialOutput=0  VectorParamsAs1DForOutWhenUnconnected=off
  wires:
  Delay2/1 -> Relational Operator1/2
  Delay/1 -> Add/2
  Relational Operator1/1 -> Delay/2
  Data Type Conversion/1 -> Add/1
  Data Type Conversion1/1 -> Out1/1
  SendFlag/1 -> Data Type Conversion/1, Switch/1
  Constant1/1 -> Switch/3
  Switch/1 -> Data Type Conversion1/1
  Relational Operator/1 -> Switch/2
  MsgLstCnt/1 -> Relational Operator1/1, Delay2/1, Relational Operator/2
  Add/1 -> Relational Operator/1, Delay/1

== system EHB_speedgoat_R2020a_V1/保留/TIF_01/YS4020_M_2/YS4020_M/FIU_CH1/Protect ==
  KL30_In : Inport
  KL31_In : Inport  Port=2
  COM_In : Inport  Port=3
  Open_In : Inport  Port=4
  Compare To Constant{,2,12,14} (4 alike) : simulink/Logic and Bit Operations/Compare To Constant  relop===  const=1  OutDataTypeStr=boolean
  Compare To Constant{1,3..11,13,15} (12 alike) : simulink/Logic and Bit Operations/Compare To Constant  relop===  const=0  OutDataTypeStr=boolean
  Logical Operator{,1..3} (4 alike) : Logic  Inputs=4  AllPortsSameDT=off  OutDataTypeStr=boolean
  KL30_Out : Outport
  KL31_Out : Outport  Port=2
  COM_Out : Outport  Port=3
  Open_Out : Outport  Port=4
  wires:
  [Open_In] -> Compare To Constant14/1
  [COM_In] -> Compare To Constant13/1
  [KL31_In] -> Compare To Constant10/1
  [KL30_In] -> Compare To Constant8/1
  [Open_In] -> Compare To Constant15/1
  [COM_In] -> Compare To Constant12/1
  [KL31_In] -> Compare To Constant11/1
  [KL30_In] -> Compare To Constant7/1
  [COM_In] -> Compare To Constant5/1
  [KL31_In] -> Compare To Constant2/1
  [KL30_In] -> Compare To Constant1/1
  [Open_In] -> Compare To Constant6/1
  [COM_In] -> Compare To Constant4/1
  [KL31_In] -> Compare To Constant3/1
  [KL30_In] -> Compare To Constant/1
  [Open_In] -> Compare To Constant9/1
  Logical Operator/1 -> [KL30_Out]
  Logical Operator3/1 -> [Open_Out]
  Logical Operator2/1 -> [COM_Out]
  Logical Operator1/1 -> [KL31_Out]
  [Open_Out] -> Open_Out/1
  Compare To Constant7/1 -> Logical Operator2/1
  Compare To Constant11/1 -> Logical Operator2/2
  Compare To Constant12/1 -> Logical Operator2/3
  Compare To Constant15/1 -> Logical Operator2/4
  Compare To Constant14/1 -> Logical Operator3/4
  Compare To Constant13/1 -> Logical Operator3/3
  Compare To Constant10/1 -> Logical Operator3/2
  Compare To Constant8/1 -> Logical Operator3/1
  Compare To Constant1/1 -> Logical Operator1/1
  Compare To Constant2/1 -> Logical Operator1/2
  Compare To Constant5/1 -> Logical Operator1/3
  Compare To Constant6/1 -> Logical Operator1/4
  Compare To Constant9/1 -> Logical Operator/4
  Open_In/1 -> [Open_In]
  [KL31_Out] -> KL31_Out/1
  [KL30_Out] -> KL30_Out/1
  [COM_Out] -> COM_Out/1
  Compare To Constant4/1 -> Logical Operator/3
  Compare To Constant3/1 -> Logical Operator/2
  KL31_In/1 -> [KL31_In]
  KL30_In/1 -> [KL30_In]
  COM_In/1 -> [COM_In]
  Compare To Constant/1 -> Logical Operator/1

== system EHB_speedgoat_R2020a_V1/保留/TIF_01/YS4020_M_2/YS4020_M/FIU_CH10/Protect ==
  KL30_In : Inport
  KL31_In : Inport  Port=2
  COM_In : Inport  Port=3
  Open_In : Inport  Port=4
  Compare To Constant{,2,12,14} (4 alike) : simulink/Logic and Bit Operations/Compare To Constant  relop===  const=1  OutDataTypeStr=boolean
  Compare To Constant{1,3..11,13,15} (12 alike) : simulink/Logic and Bit Operations/Compare To Constant  relop===  const=0  OutDataTypeStr=boolean
  Logical Operator{,1..3} (4 alike) : Logic  Inputs=4  AllPortsSameDT=off  OutDataTypeStr=boolean
  KL30_Out : Outport
  KL31_Out : Outport  Port=2
  COM_Out : Outport  Port=3
  Open_Out : Outport  Port=4
  wires:
  Compare To Constant/1 -> Logical Operator/1
  COM_In/1 -> [COM_In]
  KL30_In/1 -> [KL30_In]
  KL31_In/1 -> [KL31_In]
  Compare To Constant3/1 -> Logical Operator/2
  Compare To Constant4/1 -> Logical Operator/3
  [COM_Out] -> COM_Out/1
  [KL30_Out] -> KL30_Out/1
  [KL31_Out] -> KL31_Out/1
  Open_In/1 -> [Open_In]
  Compare To Constant9/1 -> Logical Operator/4
  Compare To Constant6/1 -> Logical Operator1/4
  Compare To Constant5/1 -> Logical Operator1/3
  Compare To Constant2/1 -> Logical Operator1/2
  Compare To Constant1/1 -> Logical Operator1/1
  Compare To Constant8/1 -> Logical Operator3/1
  Compare To Constant10/1 -> Logical Operator3/2
  Compare To Constant13/1 -> Logical Operator3/3
  Compare To Constant14/1 -> Logical Operator3/4
  Compare To Constant15/1 -> Logical Operator2/4
  Compare To Constant12/1 -> Logical Operator2/3
  Compare To Constant11/1 -> Logical Operator2/2
  Compare To Constant7/1 -> Logical Operator2/1
  [Open_Out] -> Open_Out/1
  Logical Operator1/1 -> [KL31_Out]
  Logical Operator2/1 -> [COM_Out]
  Logical Operator3/1 -> [Open_Out]
  Logical Operator/1 -> [KL30_Out]
  [Open_In] -> Compare To Constant9/1
  [KL30_In] -> Compare To Constant/1
  [KL31_In] -> Compare To Constant3/1
  [COM_In] -> Compare To Constant4/1
  [Open_In] -> Compare To Constant6/1
  [KL30_In] -> Compare To Constant1/1
  [KL31_In] -> Compare To Constant2/1
  [COM_In] -> Compare To Constant5/1
  [KL30_In] -> Compare To Constant7/1
  [KL31_In] -> Compare To Constant11/1
  [COM_In] -> Compare To Constant12/1
  [Open_In] -> Compare To Constant15/1
  [KL30_In] -> Compare To Constant8/1
  [KL31_In] -> Compare To Constant10/1
  [COM_In] -> Compare To Constant13/1
  [Open_In] -> Compare To Constant14/1

== system EHB_speedgoat_R2020a_V1/保留/TIF_01/YS4020_M_2/YS4020_M/FIU_CH11/Protect ==
  KL30_In : Inport
  KL31_In : Inport  Port=2
  COM_In : Inport  Port=3
  Open_In : Inport  Port=4
  Compare To Constant{,2,12,14} (4 alike) : simulink/Logic and Bit Operations/Compare To Constant  relop===  const=1  OutDataTypeStr=boolean
  Compare To Constant{1,3..11,13,15} (12 alike) : simulink/Logic and Bit Operations/Compare To Constant  relop===  const=0  OutDataTypeStr=boolean
  Logical Operator{,1..3} (4 alike) : Logic  Inputs=4  AllPortsSameDT=off  OutDataTypeStr=boolean
  KL30_Out : Outport
  KL31_Out : Outport  Port=2
  COM_Out : Outport  Port=3
  Open_Out : Outport  Port=4
  wires:
  Compare To Constant/1 -> Logical Operator/1
  COM_In/1 -> [COM_In]
  KL30_In/1 -> [KL30_In]
  KL31_In/1 -> [KL31_In]
  Compare To Constant3/1 -> Logical Operator/2
  Compare To Constant4/1 -> Logical Operator/3
  [COM_Out] -> COM_Out/1
  [KL30_Out] -> KL30_Out/1
  [KL31_Out] -> KL31_Out/1
  Open_In/1 -> [Open_In]
  Compare To Constant9/1 -> Logical Operator/4
  Compare To Constant6/1 -> Logical Operator1/4
  Compare To Constant5/1 -> Logical Operator1/3
  Compare To Constant2/1 -> Logical Operator1/2
  Compare To Constant1/1 -> Logical Operator1/1
  Compare To Constant8/1 -> Logical Operator3/1
  Compare To Constant10/1 -> Logical Operator3/2
  Compare To Constant13/1 -> Logical Operator3/3
  Compare To Constant14/1 -> Logical Operator3/4
  Compare To Constant15/1 -> Logical Operator2/4
  Compare To Constant12/1 -> Logical Operator2/3
  Compare To Constant11/1 -> Logical Operator2/2
  Compare To Constant7/1 -> Logical Operator2/1
  [Open_Out] -> Open_Out/1
  Logical Operator1/1 -> [KL31_Out]
  Logical Operator2/1 -> [COM_Out]
  Logical Operator3/1 -> [Open_Out]
  Logical Operator/1 -> [KL30_Out]
  [Open_In] -> Compare To Constant9/1
  [KL30_In] -> Compare To Constant/1
  [KL31_In] -> Compare To Constant3/1
  [COM_In] -> Compare To Constant4/1
  [Open_In] -> Compare To Constant6/1
  [KL30_In] -> Compare To Constant1/1
  [KL31_In] -> Compare To Constant2/1
  [COM_In] -> Compare To Constant5/1
  [KL30_In] -> Compare To Constant7/1
  [KL31_In] -> Compare To Constant11/1
  [COM_In] -> Compare To Constant12/1
  [Open_In] -> Compare To Constant15/1
  [KL30_In] -> Compare To Constant8/1
  [KL31_In] -> Compare To Constant10/1
  [COM_In] -> Compare To Constant13/1
  [Open_In] -> Compare To Constant14/1

== system EHB_speedgoat_R2020a_V1/保留/TIF_01/YS4020_M_2/YS4020_M/FIU_CH12/Protect ==
  KL30_In : Inport
  KL31_In : Inport  Port=2
  COM_In : Inport  Port=3
  Open_In : Inport  Port=4
  Compare To Constant{,2,12,14} (4 alike) : simulink/Logic and Bit Operations/Compare To Constant  relop===  const=1  OutDataTypeStr=boolean
  Compare To Constant{1,3..11,13,15} (12 alike) : simulink/Logic and Bit Operations/Compare To Constant  relop===  const=0  OutDataTypeStr=boolean
  Logical Operator{,1..3} (4 alike) : Logic  Inputs=4  AllPortsSameDT=off  OutDataTypeStr=boolean
  KL30_Out : Outport
  KL31_Out : Outport  Port=2
  COM_Out : Outport  Port=3
  Open_Out : Outport  Port=4
  wires:
  [Open_In] -> Compare To Constant14/1
  [COM_In] -> Compare To Constant13/1
  [KL31_In] -> Compare To Constant10/1
  [KL30_In] -> Compare To Constant8/1
  [Open_In] -> Compare To Constant15/1
  [COM_In] -> Compare To Constant12/1
  [KL31_In] -> Compare To Constant11/1
  [KL30_In] -> Compare To Constant7/1
  [COM_In] -> Compare To Constant5/1
  [KL31_In] -> Compare To Constant2/1
  [KL30_In] -> Compare To Constant1/1
  [Open_In] -> Compare To Constant6/1
  [COM_In] -> Compare To Constant4/1
  [KL31_In] -> Compare To Constant3/1
  [KL30_In] -> Compare To Constant/1
  [Open_In] -> Compare To Constant9/1
  Logical Operator/1 -> [KL30_Out]
  Logical Operator3/1 -> [Open_Out]
  Logical Operator2/1 -> [COM_Out]
  Logical Operator1/1 -> [KL31_Out]
  [Open_Out] -> Open_Out/1
  Compare To Constant7/1 -> Logical Operator2/1
  Compare To Constant11/1 -> Logical Operator2/2
  Compare To Constant12/1 -> Logical Operator2/3
  Compare To Constant15/1 -> Logical Operator2/4
  Compare To Constant14/1 -> Logical Operator3/4
  Compare To Constant13/1 -> Logical Operator3/3
  Compare To Constant10/1 -> Logical Operator3/2
  Compare To Constant8/1 -> Logical Operator3/1
  Compare To Constant1/1 -> Logical Operator1/1
  Compare To Constant2/1 -> Logical Operator1/2
  Compare To Constant5/1 -> Logical Operator1/3
  Compare To Constant6/1 -> Logical Operator1/4
  Compare To Constant9/1 -> Logical Operator/4
  Open_In/1 -> [Open_In]
  [KL31_Out] -> KL31_Out/1
  [KL30_Out] -> KL30_Out/1
  [COM_Out] -> COM_Out/1
  Compare To Constant4/1 -> Logical Operator/3
  Compare To Constant3/1 -> Logical Operator/2
  KL31_In/1 -> [KL31_In]
  KL30_In/1 -> [KL30_In]
  COM_In/1 -> [COM_In]
  Compare To Constant/1 -> Logical Operator/1

== system EHB_speedgoat_R2020a_V1/保留/TIF_01/YS4020_M_2/YS4020_M/FIU_CH13/Protect ==
  KL30_In : Inport
  KL31_In : Inport  Port=2
  COM_In : Inport  Port=3
  Open_In : Inport  Port=4
  Compare To Constant{,2,12,14} (4 alike) : simulink/Logic and Bit Operations/Compare To Constant  relop===  const=1  OutDataTypeStr=boolean
  Compare To Constant{1,3..11,13,15} (12 alike) : simulink/Logic and Bit Operations/Compare To Constant  relop===  const=0  OutDataTypeStr=boolean
  Logical Operator{,1..3} (4 alike) : Logic  Inputs=4  AllPortsSameDT=off  OutDataTypeStr=boolean
  KL30_Out : Outport
  KL31_Out : Outport  Port=2
  COM_Out : Outport  Port=3
  Open_Out : Outport  Port=4
  wires:
  [Open_In] -> Compare To Constant14/1
  [COM_In] -> Compare To Constant13/1
  [KL31_In] -> Compare To Constant10/1
  [KL30_In] -> Compare To Constant8/1
  [Open_In] -> Compare To Constant15/1
  [COM_In] -> Compare To Constant12/1
  [KL31_In] -> Compare To Constant11/1
  [KL30_In] -> Compare To Constant7/1
  [COM_In] -> Compare To Constant5/1
  [KL31_In] -> Compare To Constant2/1
  [KL30_In] -> Compare To Constant1/1
  [Open_In] -> Compare To Constant6/1
  [COM_In] -> Compare To Constant4/1
  [KL31_In] -> Compare To Constant3/1
  [KL30_In] -> Compare To Constant/1
  [Open_In] -> Compare To Constant9/1
  Logical Operator/1 -> [KL30_Out]
  Logical Operator3/1 -> [Open_Out]
  Logical Operator2/1 -> [COM_Out]
  Logical Operator1/1 -> [KL31_Out]
  [Open_Out] -> Open_Out/1
  Compare To Constant7/1 -> Logical Operator2/1
  Compare To Constant11/1 -> Logical Operator2/2
  Compare To Constant12/1 -> Logical Operator2/3
  Compare To Constant15/1 -> Logical Operator2/4
  Compare To Constant14/1 -> Logical Operator3/4
  Compare To Constant13/1 -> Logical Operator3/3
  Compare To Constant10/1 -> Logical Operator3/2
  Compare To Constant8/1 -> Logical Operator3/1
  Compare To Constant1/1 -> Logical Operator1/1
  Compare To Constant2/1 -> Logical Operator1/2
  Compare To Constant5/1 -> Logical Operator1/3
  Compare To Constant6/1 -> Logical Operator1/4
  Compare To Constant9/1 -> Logical Operator/4
  Open_In/1 -> [Open_In]
  [KL31_Out] -> KL31_Out/1
  [KL30_Out] -> KL30_Out/1
  [COM_Out] -> COM_Out/1
  Compare To Constant4/1 -> Logical Operator/3
  Compare To Constant3/1 -> Logical Operator/2
  KL31_In/1 -> [KL31_In]
  KL30_In/1 -> [KL30_In]
  COM_In/1 -> [COM_In]
  Compare To Constant/1 -> Logical Operator/1

== system EHB_speedgoat_R2020a_V1/保留/TIF_01/YS4020_M_2/YS4020_M/FIU_CH14/Protect ==
  KL30_In : Inport
  KL31_In : Inport  Port=2
  COM_In : Inport  Port=3
  Open_In : Inport  Port=4
  Compare To Constant{,2,12,14} (4 alike) : simulink/Logic and Bit Operations/Compare To Constant  relop===  const=1  OutDataTypeStr=boolean
  Compare To Constant{1,3..11,13,15} (12 alike) : simulink/Logic and Bit Operations/Compare To Constant  relop===  const=0  OutDataTypeStr=boolean
  Logical Operator{,1..3} (4 alike) : Logic  Inputs=4  AllPortsSameDT=off  OutDataTypeStr=boolean
  KL30_Out : Outport
  KL31_Out : Outport  Port=2
  COM_Out : Outport  Port=3
  Open_Out : Outport  Port=4
  wires:
  Compare To Constant/1 -> Logical Operator/1
  COM_In/1 -> [COM_In]
  KL30_In/1 -> [KL30_In]
  KL31_In/1 -> [KL31_In]
  Compare To Constant3/1 -> Logical Operator/2
  Compare To Constant4/1 -> Logical Operator/3
  [COM_Out] -> COM_Out/1
  [KL30_Out] -> KL30_Out/1
  [KL31_Out] -> KL31_Out/1
  Open_In/1 -> [Open_In]
  Compare To Constant9/1 -> Logical Operator/4
  Compare To Constant6/1 -> Logical Operator1/4
  Compare To Constant5/1 -> Logical Operator1/3
  Compare To Constant2/1 -> Logical Operator1/2
  Compare To Constant1/1 -> Logical Operator1/1
  Compare To Constant8/1 -> Logical Operator3/1
  Compare To Constant10/1 -> Logical Operator3/2
  Compare To Constant13/1 -> Logical Operator3/3
  Compare To Constant14/1 -> Logical Operator3/4
  Compare To Constant15/1 -> Logical Operator2/4
  Compare To Constant12/1 -> Logical Operator2/3
  Compare To Constant11/1 -> Logical Operator2/2
  Compare To Constant7/1 -> Logical Operator2/1
  [Open_Out] -> Open_Out/1
  Logical Operator1/1 -> [KL31_Out]
  Logical Operator2/1 -> [COM_Out]
  Logical Operator3/1 -> [Open_Out]
  Logical Operator/1 -> [KL30_Out]
  [Open_In] -> Compare To Constant9/1
  [KL30_In] -> Compare To Constant/1
  [KL31_In] -> Compare To Constant3/1
  [COM_In] -> Compare To Constant4/1
  [Open_In] -> Compare To Constant6/1
  [KL30_In] -> Compare To Constant1/1
  [KL31_In] -> Compare To Constant2/1
  [COM_In] -> Compare To Constant5/1
  [KL30_In] -> Compare To Constant7/1
  [KL31_In] -> Compare To Constant11/1
  [COM_In] -> Compare To Constant12/1
  [Open_In] -> Compare To Constant15/1
  [KL30_In] -> Compare To Constant8/1
  [KL31_In] -> Compare To Constant10/1
  [COM_In] -> Compare To Constant13/1
  [Open_In] -> Compare To Constant14/1

== system EHB_speedgoat_R2020a_V1/保留/TIF_01/YS4020_M_2/YS4020_M/FIU_CH15/Protect ==
  KL30_In : Inport
  KL31_In : Inport  Port=2
  COM_In : Inport  Port=3
  Open_In : Inport  Port=4
  Compare To Constant{,2,12,14} (4 alike) : simulink/Logic and Bit Operations/Compare To Constant  relop===  const=1  OutDataTypeStr=boolean
  Compare To Constant{1,3..11,13,15} (12 alike) : simulink/Logic and Bit Operations/Compare To Constant  relop===  const=0  OutDataTypeStr=boolean
  Logical Operator{,1..3} (4 alike) : Logic  Inputs=4  AllPortsSameDT=off  OutDataTypeStr=boolean
  KL30_Out : Outport
  KL31_Out : Outport  Port=2
  COM_Out : Outport  Port=3
  Open_Out : Outport  Port=4
  wires:
  [Open_In] -> Compare To Constant14/1
  [COM_In] -> Compare To Constant13/1
  [KL31_In] -> Compare To Constant10/1
  [KL30_In] -> Compare To Constant8/1
  [Open_In] -> Compare To Constant15/1
  [COM_In] -> Compare To Constant12/1
  [KL31_In] -> Compare To Constant11/1
  [KL30_In] -> Compare To Constant7/1
  [COM_In] -> Compare To Constant5/1
  [KL31_In] -> Compare To Constant2/1
  [KL30_In] -> Compare To Constant1/1
  [Open_In] -> Compare To Constant6/1
  [COM_In] -> Compare To Constant4/1
  [KL31_In] -> Compare To Constant3/1
  [KL30_In] -> Compare To Constant/1
  [Open_In] -> Compare To Constant9/1
  Logical Operator/1 -> [KL30_Out]
  Logical Operator3/1 -> [Open_Out]
  Logical Operator2/1 -> [COM_Out]
  Logical Operator1/1 -> [KL31_Out]
  [Open_Out] -> Open_Out/1
  Compare To Constant7/1 -> Logical Operator2/1
  Compare To Constant11/1 -> Logical Operator2/2
  Compare To Constant12/1 -> Logical Operator2/3
  Compare To Constant15/1 -> Logical Operator2/4
  Compare To Constant14/1 -> Logical Operator3/4
  Compare To Constant13/1 -> Logical Operator3/3
  Compare To Constant10/1 -> Logical Operator3/2
  Compare To Constant8/1 -> Logical Operator3/1
  Compare To Constant1/1 -> Logical Operator1/1
  Compare To Constant2/1 -> Logical Operator1/2
  Compare To Constant5/1 -> Logical Operator1/3
  Compare To Constant6/1 -> Logical Operator1/4
  Compare To Constant9/1 -> Logical Operator/4
  Open_In/1 -> [Open_In]
  [KL31_Out] -> KL31_Out/1
  [KL30_Out] -> KL30_Out/1
  [COM_Out] -> COM_Out/1
  Compare To Constant4/1 -> Logical Operator/3
  Compare To Constant3/1 -> Logical Operator/2
  KL31_In/1 -> [KL31_In]
  KL30_In/1 -> [KL30_In]
  COM_In/1 -> [COM_In]
  Compare To Constant/1 -> Logical Operator/1

== system EHB_speedgoat_R2020a_V1/保留/TIF_01/YS4020_M_2/YS4020_M/FIU_CH16/Protect ==
  KL30_In : Inport
  KL31_In : Inport  Port=2
  COM_In : Inport  Port=3
  Open_In : Inport  Port=4
  Compare To Constant{,2,12,14} (4 alike) : simulink/Logic and Bit Operations/Compare To Constant  relop===  const=1  OutDataTypeStr=boolean
  Compare To Constant{1,3..11,13,15} (12 alike) : simulink/Logic and Bit Operations/Compare To Constant  relop===  const=0  OutDataTypeStr=boolean
  Logical Operator{,1..3} (4 alike) : Logic  Inputs=4  AllPortsSameDT=off  OutDataTypeStr=boolean
  KL30_Out : Outport
  KL31_Out : Outport  Port=2
  COM_Out : Outport  Port=3
  Open_Out : Outport  Port=4
  wires:
  Compare To Constant/1 -> Logical Operator/1
  COM_In/1 -> [COM_In]
  KL30_In/1 -> [KL30_In]
  KL31_In/1 -> [KL31_In]
  Compare To Constant3/1 -> Logical Operator/2
  Compare To Constant4/1 -> Logical Operator/3
  [COM_Out] -> COM_Out/1
  [KL30_Out] -> KL30_Out/1
  [KL31_Out] -> KL31_Out/1
  Open_In/1 -> [Open_In]
  Compare To Constant9/1 -> Logical Operator/4
  Compare To Constant6/1 -> Logical Operator1/4
  Compare To Constant5/1 -> Logical Operator1/3
  Compare To Constant2/1 -> Logical Operator1/2
  Compare To Constant1/1 -> Logical Operator1/1
  Compare To Constant8/1 -> Logical Operator3/1
  Compare To Constant10/1 -> Logical Operator3/2
  Compare To Constant13/1 -> Logical Operator3/3
  Compare To Constant14/1 -> Logical Operator3/4
  Compare To Constant15/1 -> Logical Operator2/4
  Compare To Constant12/1 -> Logical Operator2/3
  Compare To Constant11/1 -> Logical Operator2/2
  Compare To Constant7/1 -> Logical Operator2/1
  [Open_Out] -> Open_Out/1
  Logical Operator1/1 -> [KL31_Out]
  Logical Operator2/1 -> [COM_Out]
  Logical Operator3/1 -> [Open_Out]
  Logical Operator/1 -> [KL30_Out]
  [Open_In] -> Compare To Constant9/1
  [KL30_In] -> Compare To Constant/1
  [KL31_In] -> Compare To Constant3/1
  [COM_In] -> Compare To Constant4/1
  [Open_In] -> Compare To Constant6/1
  [KL30_In] -> Compare To Constant1/1
  [KL31_In] -> Compare To Constant2/1
  [COM_In] -> Compare To Constant5/1
  [KL30_In] -> Compare To Constant7/1
  [KL31_In] -> Compare To Constant11/1
  [COM_In] -> Compare To Constant12/1
  [Open_In] -> Compare To Constant15/1
  [KL30_In] -> Compare To Constant8/1
  [KL31_In] -> Compare To Constant10/1
  [COM_In] -> Compare To Constant13/1
  [Open_In] -> Compare To Constant14/1

== system EHB_speedgoat_R2020a_V1/保留/TIF_01/YS4020_M_2/YS4020_M/FIU_CH17/Protect ==
  KL30_In : Inport
  KL31_In : Inport  Port=2
  COM_In : Inport  Port=3
  Open_In : Inport  Port=4
  Compare To Constant{,2,12,14} (4 alike) : simulink/Logic and Bit Operations/Compare To Constant  relop===  const=1  OutDataTypeStr=boolean
  Compare To Constant{1,3..11,13,15} (12 alike) : simulink/Logic and Bit Operations/Compare To Constant  relop===  const=0  OutDataTypeStr=boolean
  Logical Operator{,1..3} (4 alike) : Logic  Inputs=4  AllPortsSameDT=off  OutDataTypeStr=boolean
  KL30_Out : Outport
  KL31_Out : Outport  Port=2
  COM_Out : Outport  Port=3
  Open_Out : Outport  Port=4
  wires:
  [Open_In] -> Compare To Constant14/1
  [COM_In] -> Compare To Constant13/1
  [KL31_In] -> Compare To Constant10/1
  [KL30_In] -> Compare To Constant8/1
  [Open_In] -> Compare To Constant15/1
  [COM_In] -> Compare To Constant12/1
  [KL31_In] -> Compare To Constant11/1
  [KL30_In] -> Compare To Constant7/1
  [COM_In] -> Compare To Constant5/1
  [KL31_In] -> Compare To Constant2/1
  [KL30_In] -> Compare To Constant1/1
  [Open_In] -> Compare To Constant6/1
  [COM_In] -> Compare To Constant4/1
  [KL31_In] -> Compare To Constant3/1
  [KL30_In] -> Compare To Constant/1
  [Open_In] -> Compare To Constant9/1
  Logical Operator/1 -> [KL30_Out]
  Logical Operator3/1 -> [Open_Out]
  Logical Operator2/1 -> [COM_Out]
  Logical Operator1/1 -> [KL31_Out]
  [Open_Out] -> Open_Out/1
  Compare To Constant7/1 -> Logical Operator2/1
  Compare To Constant11/1 -> Logical Operator2/2
  Compare To Constant12/1 -> Logical Operator2/3
  Compare To Constant15/1 -> Logical Operator2/4
  Compare To Constant14/1 -> Logical Operator3/4
  Compare To Constant13/1 -> Logical Operator3/3
  Compare To Constant10/1 -> Logical Operator3/2
  Compare To Constant8/1 -> Logical Operator3/1
  Compare To Constant1/1 -> Logical Operator1/1
  Compare To Constant2/1 -> Logical Operator1/2
  Compare To Constant5/1 -> Logical Operator1/3
  Compare To Constant6/1 -> Logical Operator1/4
  Compare To Constant9/1 -> Logical Operator/4
  Open_In/1 -> [Open_In]
  [KL31_Out] -> KL31_Out/1
  [KL30_Out] -> KL30_Out/1
  [COM_Out] -> COM_Out/1
  Compare To Constant4/1 -> Logical Operator/3
  Compare To Constant3/1 -> Logical Operator/2
  KL31_In/1 -> [KL31_In]
  KL30_In/1 -> [KL30_In]
  COM_In/1 -> [COM_In]
  Compare To Constant/1 -> Logical Operator/1

== system EHB_speedgoat_R2020a_V1/保留/TIF_01/YS4020_M_2/YS4020_M/FIU_CH18/Protect ==
  KL30_In : Inport
  KL31_In : Inport  Port=2
  COM_In : Inport  Port=3
  Open_In : Inport  Port=4
  Compare To Constant{,2,12,14} (4 alike) : simulink/Logic and Bit Operations/Compare To Constant  relop===  const=1  OutDataTypeStr=boolean
  Compare To Constant{1,3..11,13,15} (12 alike) : simulink/Logic and Bit Operations/Compare To Constant  relop===  const=0  OutDataTypeStr=boolean
  Logical Operator{,1..3} (4 alike) : Logic  Inputs=4  AllPortsSameDT=off  OutDataTypeStr=boolean
  KL30_Out : Outport
  KL31_Out : Outport  Port=2
  COM_Out : Outport  Port=3
  Open_Out : Outport  Port=4
  wires:
  Compare To Constant/1 -> Logical Operator/1
  COM_In/1 -> [COM_In]
  KL30_In/1 -> [KL30_In]
  KL31_In/1 -> [KL31_In]
  Compare To Constant3/1 -> Logical Operator/2
  Compare To Constant4/1 -> Logical Operator/3
  [COM_Out] -> COM_Out/1
  [KL30_Out] -> KL30_Out/1
  [KL31_Out] -> KL31_Out/1
  Open_In/1 -> [Open_In]
  Compare To Constant9/1 -> Logical Operator/4
  Compare To Constant6/1 -> Logical Operator1/4
  Compare To Constant5/1 -> Logical Operator1/3
  Compare To Constant2/1 -> Logical Operator1/2
  Compare To Constant1/1 -> Logical Operator1/1
  Compare To Constant8/1 -> Logical Operator3/1
  Compare To Constant10/1 -> Logical Operator3/2
  Compare To Constant13/1 -> Logical Operator3/3
  Compare To Constant14/1 -> Logical Operator3/4
  Compare To Constant15/1 -> Logical Operator2/4
  Compare To Constant12/1 -> Logical Operator2/3
  Compare To Constant11/1 -> Logical Operator2/2
  Compare To Constant7/1 -> Logical Operator2/1
  [Open_Out] -> Open_Out/1
  Logical Operator1/1 -> [KL31_Out]
  Logical Operator2/1 -> [COM_Out]
  Logical Operator3/1 -> [Open_Out]
  Logical Operator/1 -> [KL30_Out]
  [Open_In] -> Compare To Constant9/1
  [KL30_In] -> Compare To Constant/1
  [KL31_In] -> Compare To Constant3/1
  [COM_In] -> Compare To Constant4/1
  [Open_In] -> Compare To Constant6/1
  [KL30_In] -> Compare To Constant1/1
  [KL31_In] -> Compare To Constant2/1
  [COM_In] -> Compare To Constant5/1
  [KL30_In] -> Compare To Constant7/1
  [KL31_In] -> Compare To Constant11/1
  [COM_In] -> Compare To Constant12/1
  [Open_In] -> Compare To Constant15/1
  [KL30_In] -> Compare To Constant8/1
  [KL31_In] -> Compare To Constant10/1
  [COM_In] -> Compare To Constant13/1
  [Open_In] -> Compare To Constant14/1
